simulink model "Glucose_model_Final"  (R2022b)
settings: Solver=VariableStepAuto  StartTime=0.0  StopTime=1000  RelTol=1e-3
values from neighbouring files (symbols this model uses):
  G_0 = 12000    [main_Parameters_IntialCondition_plots.m]
  h_10 = 0.1    [main_Parameters_IntialCondition_plots.m]
  h_20 = 0.2    [main_Parameters_IntialCondition_plots.m]
  h_30 = 0.1    [main_Parameters_IntialCondition_plots.m]
  Ii_0 = 220    [main_Parameters_IntialCondition_plots.m]
  Ip_0 = 90    [main_Parameters_IntialCondition_plots.m]
  td = p.td    [Compute_Fixed_point.m]    (also in Linearization_method.m; main_Parameters_IntialCondition_plots.m = 36)
  ti = p.ti    [Compute_Fixed_point.m]    (also in Linearization_method.m; main_Parameters_IntialCondition_plots.m = 100)
  tp = p.tp    [Compute_Fixed_point.m]    (also in Linearization_method.m; main_Parameters_IntialCondition_plots.m = 6)
settings Model: Creator=ramma  LastModifiedBy=hayden
settings DebuggingCC: UnconnectedInputMsg=warning  UnconnectedOutputMsg=warning  UnconnectedLineMsg=warning
settings ModelReferenceCC: EnableRefExpFcnMdlSchedulingChecks=on
settings RTWCC: DLArmComputeVersion=19.05

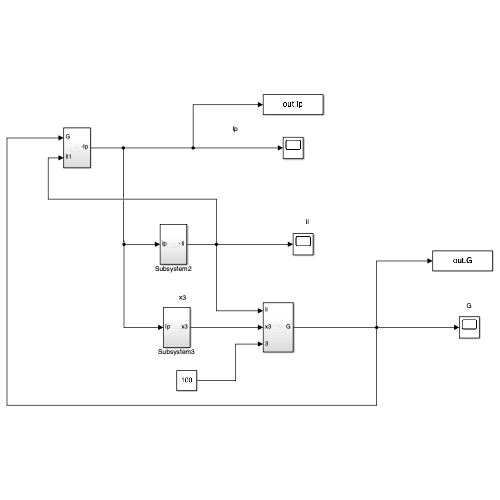
[thumbnail: Simulink's stored preview of the top-level diagram]
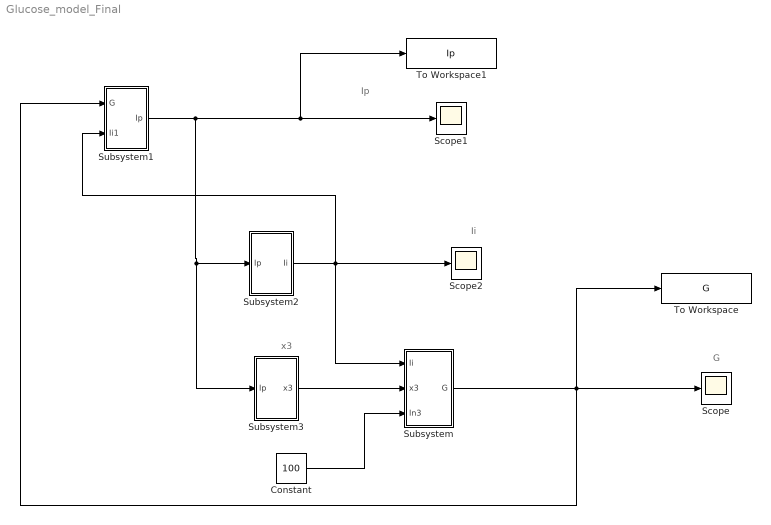
== system Glucose_model_Final ==
  note: G
  note: Ii
  note: Ip
  note: x3
  Constant : Constant  Value=100
  Scope : Scope
  Scope1 : Scope
  Scope2 : Scope
  Subsystem : Subsystem
  Subsystem1 : Subsystem
  Subsystem2 : Subsystem
  Subsystem3 : Subsystem
  To Workspace : ToWorkspace  VariableName=G  SampleTime=-1
      settings: Save2DSignal=2-D array (concatenate along first dimension)
  To Workspace1 : ToWorkspace  VariableName=Ip  SampleTime=-1
      settings: Save2DSignal=2-D array (concatenate along first dimension)
  wires:
  Subsystem2/1(Ii) -> Subsystem/1(Ii), Subsystem1/2(Ii1), Scope2/1
  Subsystem/1(G) -> To Workspace/1, Scope/1, Subsystem1/1(G)
  Constant/1 -> Subsystem/3(In3)
  Subsystem3/1(x3) -> Subsystem/2(x3)
  Subsystem1/1(Ip) -> To Workspace1/1, Scope1/1, Subsystem3/1(Ip), Subsystem2/1(Ip)

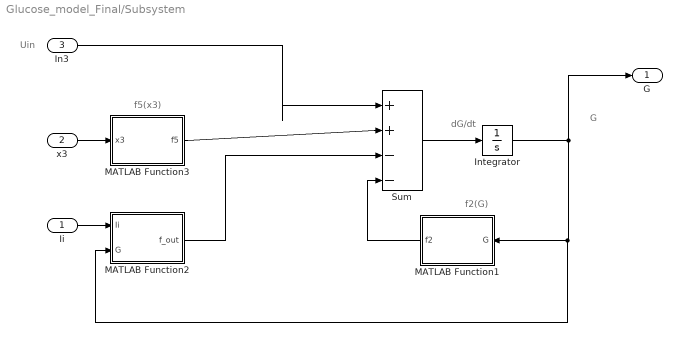
== system Glucose_model_Final/Subsystem ==
  note: f5(x3)
  note: Uin
  note: f2(G)
  note: G
  note: dG/dt
  Ii : Inport
  x3 : Inport  Port=2
  In3 : Inport  Port=3
  Integrator : Integrator  InitialCondition=G_0
  MATLAB Function1 : MATLAB Function  TreatAsAtomicUnit=on
  MATLAB Function2 : MATLAB Function  TreatAsAtomicUnit=on
  MATLAB Function3 : MATLAB Function  TreatAsAtomicUnit=on
  Sum : Sum  Inputs=|++--
  G : Outport
  wires:
  Integrator/1 -> G/1, MATLAB Function2/2(G), MATLAB Function1/1(G)
  Sum/1 -> Integrator/1
  MATLAB Function1/1(f2) -> Sum/4
  MATLAB Function2/1(f_out) -> Sum/3
  MATLAB Function3/1(f5) -> Sum/2
  Ii/1 -> MATLAB Function2/1(Ii)
  x3/1 -> MATLAB Function3/1(x3)
  In3/1 -> Sum/1

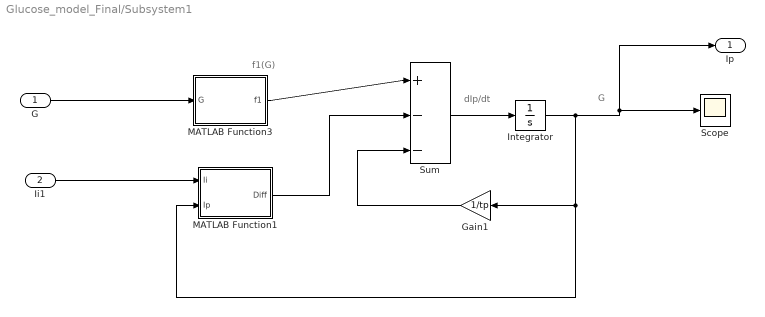
== system Glucose_model_Final/Subsystem1 ==
  note: dIp/dt
  note: G
  note: f1(G)
  G : Inport
  Ii1 : Inport  Port=2
  Gain1 : Gain  Gain=1/tp
  Integrator : Integrator  InitialCondition=Ip_0
  MATLAB Function1 : MATLAB Function  TreatAsAtomicUnit=on
  MATLAB Function3 : MATLAB Function  TreatAsAtomicUnit=on
  Scope : Scope
  Sum : Sum  Inputs=|+--
  Ip : Outport
  wires:
  MATLAB Function1/1(Diff) -> Sum/2
  MATLAB Function3/1(f1) -> Sum/1
  Integrator/1 -> MATLAB Function1/2(Ip), Gain1/1, Ip/1, Scope/1
  Ii1/1 -> MATLAB Function1/1(Ii)
  G/1 -> MATLAB Function3/1(G)
  Sum/1 -> Integrator/1
  Gain1/1 -> Sum/3

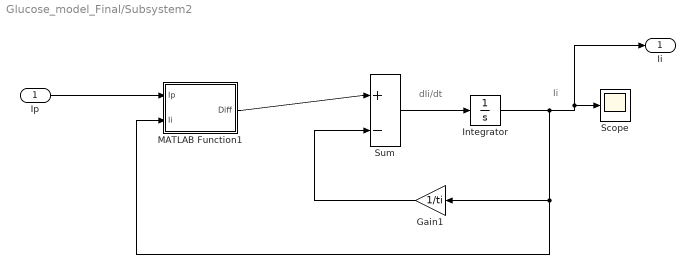
== system Glucose_model_Final/Subsystem2 ==
  note: dIi/dt
  note: Ii
  Ip : Inport
  Gain1 : Gain  Gain=1/ti
  Integrator : Integrator  InitialCondition=Ii_0
  MATLAB Function1 : MATLAB Function  TreatAsAtomicUnit=on
  Scope : Scope
  Sum : Sum  Inputs=|+-
  Ii : Outport
  wires:
  Integrator/1 -> Gain1/1, MATLAB Function1/2(Ii), Ii/1, Scope/1
  Gain1/1 -> Sum/2
  Ip/1 -> MATLAB Function1/1(Ip)
  MATLAB Function1/1(Diff) -> Sum/1
  Sum/1 -> Integrator/1

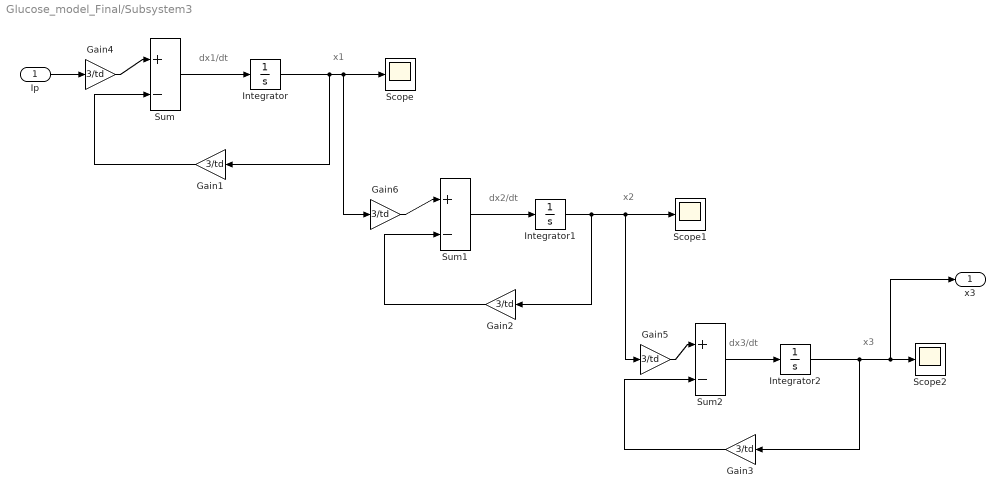
== system Glucose_model_Final/Subsystem3 ==
  note: dx1/dt
  note: x1
  note: x2
  note: dx2/dt
  note: dx3/dt
  note: x3
  Ip : Inport
  Gain{1..6} (6 alike) : Gain  Gain=3/td
  Integrator : Integrator  InitialCondition=h_10
  Integrator1 : Integrator  InitialCondition=h_20
  Integrator2 : Integrator  InitialCondition=h_30
  Scope : Scope
  Scope1 : Scope
  Scope2 : Scope
  Sum : Sum  Inputs=|+-
  Sum1 : Sum  Inputs=|+-
  Sum2 : Sum  Inputs=|+-
  x3 : Outport
  wires:
  Integrator/1 -> Gain1/1, Scope/1, Gain6/1
  Gain1/1 -> Sum/2
  Sum/1 -> Integrator/1
  Gain2/1 -> Sum1/2
  Integrator1/1 -> Scope1/1, Gain5/1, Gain2/1
  Sum1/1 -> Integrator1/1
  Integrator2/1 -> Gain3/1, x3/1, Scope2/1
  Sum2/1 -> Integrator2/1
  Gain3/1 -> Sum2/2
  Ip/1 -> Gain4/1
  Gain4/1 -> Sum/1
  Gain6/1 -> Sum1/1
  Gain5/1 -> Sum2/1

== matlab function Glucose_model_Final/Subsystem1/MATLAB Function1 ==
  data: Ii input; Diff output; Ip input
function Diff = fcn(Ii,Ip)
% Constants
Vp = 3;  %'Vp' [L] 
Vi = 11; %'Vp' [L] 
% Vg = 10; %'Vp' [L]
E = 0.2; % [L min^-1]
% tp = 6;  % min
% ti = 100;% min
% td = 36;% min
% Rm = 210;% [mU min^-1]{Lui 2008}
% % p.Rm = 21;% [mU min^-1]{Tolic 2000}
% a1 = 300; %mg/L
% C1 = 2000;% mg/L
% C2 = 144;% mg/L
% C3 = 1000;% mg/L
% C4 = 80;% mU/L
% C5 = 26;% mU/L
% Ub = 72;% mg/min
% U0 = 40;% mg/min
% Um = 940;% mg/min
% Rg = 180;% mg/min 
% alpha = 0.29;% L/mU
% beta = 1.77;
%%
Rm = 210;% [mU min^-1]{Lui 2008}
C1 = 2000;% mg/L
a1 = 300; %mg/L
%% Function f2
% f1 = Rm/(1 + exp((C1-G)/a1)); % 
%%
Diff= (Ip/Vp - Ii/Vi)*E ;

== matlab function Glucose_model_Final/Subsystem/MATLAB Function2 ==
  data: Ii input; G input; f_out output
function f_out = fcn(Ii,G)
% Constants
% Vp = 3;  %'Vp' [L] 
% Vi = 11; %'Vp' [L] 
% Vg = 10; %'Vp' [L]
% E = 0.2; % [L min^-1]
% tp = 6;  % min
% ti = 100;% min
% td = 36;% min
% Rm = 210;% [mU min^-1]{Lui 2008}
% % p.Rm = 21;% [mU min^-1]{Tolic 2000}
% a1 = 300; %mg/L
% C1 = 2000;% mg/L
% C2 = 144;% mg/L
% C3 = 1000;% mg/L
% C4 = 80;% mU/L
% C5 = 26;% mU/L
% Ub = 72;% mg/min
% U0 = 40;% mg/min
% Um = 940;% mg/min
% Rg = 180;% mg/min 
% alpha = 0.29;% L/mU
% beta = 1.77;
%% f3
% Constants
C3 = 1000;% mg/L
Vg=10;
%% Function f2
Cg=G/Vg; % concentration
f3 = Cg/C3; 
%%
C4 = 80;% mU/L
E = 0.2; % [L min^-1]
ti = 100;% min
Vi = 11; %'Vp' [L] 
U0 = 40;% mg/min
Um = 940;% mg/min
beta = 1.77;
%% Function f2
C_ref = C4*(E*ti/(E*ti + Vi));
CIi=Ii/Vi; % concentration
f4 = U0 + (Um-U0)*(CIi^beta/(CIi^beta + C_ref^beta)); %  
f_out=f3*f4;

== matlab function Glucose_model_Final/Subsystem/MATLAB Function3 ==
  data: x3 input; f5 output
function f5 = fcn(x3)
% Constants
% Vp = 3;  %'Vp' [L] 
% Vi = 11; %'Vp' [L] 
% Vg = 10; %'Vp' [L]
% E = 0.2; % [L min^-1]
% tp = 6;  % min
% ti = 100;% min
% td = 36;% min
% Rm = 210;% [mU min^-1]{Lui 2008}
% % p.Rm = 21;% [mU min^-1]{Tolic 2000}
% a1 = 300; %mg/L
% C1 = 2000;% mg/L
% C2 = 144;% mg/L
% C3 = 1000;% mg/L
% C4 = 80;% mU/L
% C5 = 26;% mU/L
% Ub = 72;% mg/min
% U0 = 40;% mg/min
% Um = 940;% mg/min
% Rg = 180;% mg/min 
% alpha = 0.29;% L/mU
% beta = 1.77;
%%
Rg = 180;% mg/min 
alpha = 0.29;% L/mU
C5 = 26;% mU/L
Vp=3;
%% Function f2
Cx3=x3/Vp;
f5 = Rg/(1+ exp(alpha*(Cx3 - C5)));

== matlab function Glucose_model_Final/Subsystem2/MATLAB Function1 ==
  data: Ip input; Ii input; Diff output
function Diff = fcn(Ip,Ii)
% Constants
Vp = 3;  %'Vp' [L] 
Vi = 11; %'Vp' [L] 
% Vg = 10; %'Vp' [L]
E = 0.2; % [L min^-1]
% tp = 6;  % min
% ti = 100;% min
% td = 36;% min
% Rm = 210;% [mU min^-1]{Lui 2008}
% % p.Rm = 21;% [mU min^-1]{Tolic 2000}
% a1 = 300; %mg/L
% C1 = 2000;% mg/L
% C2 = 144;% mg/L
% C3 = 1000;% mg/L
% C4 = 80;% mU/L
% C5 = 26;% mU/L
% Ub = 72;% mg/min
% U0 = 40;% mg/min
% Um = 940;% mg/min
% Rg = 180;% mg/min 
% alpha = 0.29;% L/mU
% beta = 1.77;
%%
Rm = 210;% [mU min^-1]{Lui 2008}
C1 = 2000;% mg/L
a1 = 300; %mg/L
%% Function f2
% f1 = Rm/(1 + exp((C1-G)/a1)); % 
%%
Diff= (Ip/Vp - Ii/Vi)*E ;

== matlab function Glucose_model_Final/Subsystem1/MATLAB Function3 ==
  data: G input; f1 output
function f1 = fcn(G)
% Constants
% Vp = 3;  %'Vp' [L] 
% Vi = 11; %'Vp' [L] 
% Vg = 10; %'Vp' [L]
% E = 0.2; % [L min^-1]
% tp = 6;  % min
% ti = 100;% min
% td = 36;% min
% Rm = 210;% [mU min^-1]{Lui 2008}
% % p.Rm = 21;% [mU min^-1]{Tolic 2000}
% a1 = 300; %mg/L
% C1 = 2000;% mg/L
% C2 = 144;% mg/L
% C3 = 1000;% mg/L
% C4 = 80;% mU/L
% C5 = 26;% mU/L
% Ub = 72;% mg/min
% U0 = 40;% mg/min
% Um = 940;% mg/min
% Rg = 180;% mg/min 
% alpha = 0.29;% L/mU
% beta = 1.77;
%%
Rm = 210;% [mU min^-1]{Lui 2008}
C1 = 2000;% mg/L
a1 = 300; %mg/L
Vg=10; % L
%% Function f2
% f1 = Rm/(1 + exp((C1-G)/a1)); % 
Cg=G/Vg;
f1 = Rm/(1 + exp((C1-Cg)/a1)); %

== matlab function Glucose_model_Final/Subsystem/MATLAB Function1 ==
  data: G input; f2 output
function f2 = fcn(G)
% Constants
% Vp = 3;  %'Vp' [L] 
% Vi = 11; %'Vp' [L] 
% Vg = 10; %'Vp' [L]
% E = 0.2; % [L min^-1]
% tp = 6;  % min
% ti = 100;% min
% td = 36;% min
% Rm = 210;% [mU min^-1]{Lui 2008}
% % p.Rm = 21;% [mU min^-1]{Tolic 2000}
% a1 = 300; %mg/L
% C1 = 2000;% mg/L
% C2 = 144;% mg/L
% C3 = 1000;% mg/L
% C4 = 80;% mU/L
% C5 = 26;% mU/L
% Ub = 72;% mg/min
% U0 = 40;% mg/min
% Um = 940;% mg/min
% Rg = 180;% mg/min 
% alpha = 0.29;% L/mU
% beta = 1.77;
%%
Ub = 72;% mg/min
C2 = 144;% mg/L
Ub = 72;% mg/min
Vg=10; %L
%% Function f2
% f2 = Ub*(1 - exp(-G/C2)); %  
%%
Cg=G/Vg;
f2 = Ub*(1 - exp(-Cg/C2)); %
